simulink model "Part_3_Template"  (R2017a)
settings: Solver=ode3  StartTime=0.0  StopTime=30  FixedStep=.001  RelTol=1e-3  EnableMultiTasking=on
libraries: dspinverses x1
settings Model: Creator=Andrew Petruska  LastModifiedBy=siddh
settings OptimizationCC: LifeSpan=inf
settings DebuggingCC: SFUnexpectedBacktrackingDiag=warning  SFNoUnconditionalDefaultTransitionDiag=warning  SFExecutionAtInitializationDiag=none
settings GRTTargetCC: TargetLangStandard=C89/C90 (ANSI)  GeneratePreprocessorConditionals=Disable all
settings ConfigComp: CovMetricSettings=dw  CovHtmlReporting=on  CovSaveCumulativeToWorkspaceVar=on  CovSaveSingleToWorkspaceVar=on  CovExternalEMLEnable=off

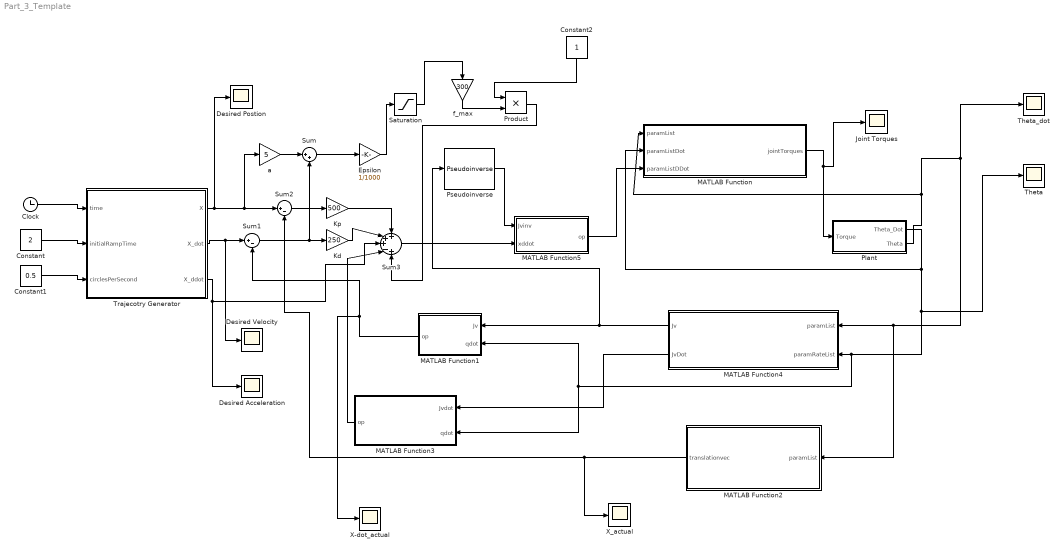
== system Part_3_Template ==
  Clock : Clock
  Constant : Constant  Value=2
  Constant1 : Constant  Value=0.5
  Constant2 : Constant
  Desired Acceleration : Scope
  Desired Postion : Scope
  Desired Velocity : Scope
  "Epsilon " : Gain  Gain=1/1000
  "Joint Torques " : Scope
  Kd : Gain  Gain=250
  Kp : Gain  Gain=500
  MATLAB Function : MATLAB Function  TreatAsAtomicUnit=on
  MATLAB Function1 : MATLAB Function  TreatAsAtomicUnit=on
  MATLAB Function2 : MATLAB Function  TreatAsAtomicUnit=on
  MATLAB Function3 : MATLAB Function  TreatAsAtomicUnit=on
  MATLAB Function4 : MATLAB Function  TreatAsAtomicUnit=on
  MATLAB Function5 : MATLAB Function  TreatAsAtomicUnit=on
  Plant : Subsystem
  Product : Product
  Pseudoinverse : dspinverses/Pseudoinverse  wanterr=off  SimulateUsing=Interpreted execution
      settings: SourceProductName=DSP System Toolbox  SourceProductBaseCode=DS
  Saturation : Saturate  UpperLimit=1  LowerLimit=-1
  Sum : Sum  Inputs=|++
  Sum1 : Sum  Inputs=|+-
  Sum2 : Sum  Inputs=|+-
  Sum3 : Sum  Inputs=+++-+
  "Theta " : Scope
  Theta_dot : Scope
  Trajecotry Generator : MATLAB Function  TreatAsAtomicUnit=on
  X-dot_actual : Scope
  X_actual : Scope
  "a " : Gain  Gain=5
  f_max : Gain  Gain=300
  wires:
  Plant/2(Theta) -> MATLAB Function2/1(paramList), MATLAB Function4/1(paramList), Theta_dot/1, MATLAB Function/1(paramList)
  Clock/1 -> Trajecotry Generator/1(time)
  Constant/1 -> Trajecotry Generator/2(initialRampTime)
  Constant1/1 -> Trajecotry Generator/3(circlesPerSecond)
  Trajecotry Generator/1(X) -> "a "/1, Sum2/1, Desired Postion/1
  Trajecotry Generator/2(X_dot) -> Sum1/1, Desired Velocity/1
  Trajecotry Generator/3(X_ddot) -> Sum3/3, Desired Acceleration/1
  Plant/1(Theta_Dot) -> MATLAB Function/2(paramListDot), MATLAB Function3/2(qdot), MATLAB Function1/2(qdot), MATLAB Function4/2(paramRateList), "Theta "/1
  MATLAB Function/1(jointTorques) -> "Joint Torques "/1, Plant/1(Torque)
  MATLAB Function4/2(JvDot) -> MATLAB Function3/1(Jvdot)
  MATLAB Function2/1(translationvec) -> X_actual/1, Sum2/2
  Sum2/1 -> Kp/1
  Kp/1 -> Sum3/1
  Sum1/1 -> Sum/2, Kd/1
  Kd/1 -> Sum3/2
  MATLAB Function3/1(op) -> Sum3/4
  MATLAB Function4/1(Jv) -> Pseudoinverse/1, MATLAB Function1/1(Jv)
  MATLAB Function1/1(op) -> X-dot_actual/1, Sum1/2
  Sum3/1 -> MATLAB Function5/2(xddot)
  Pseudoinverse/1 -> MATLAB Function5/1(Jvinv)
  MATLAB Function5/1(op) -> MATLAB Function/3(paramListDDot)
  "a "/1 -> Sum/1
  Sum/1 -> "Epsilon "/1
  "Epsilon "/1 -> Saturation/1
  Saturation/1 -> f_max/1
  f_max/1 -> Product/2
  Constant2/1 -> Product/1
  Product/1 -> Sum3/5

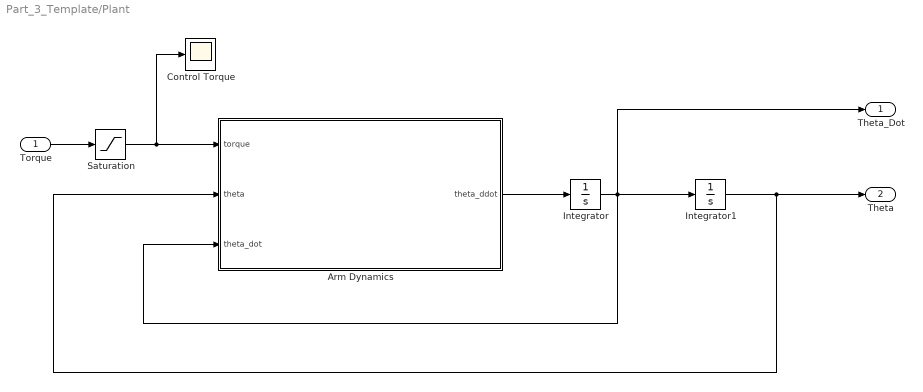
== system Part_3_Template/Plant ==
  Torque : Inport
  Arm Dynamics : MATLAB Function  TreatAsAtomicUnit=on
  Control Torque : Scope
  Integrator : Integrator  InitialCondition=[0;0;0]
  Integrator1 : Integrator  InitialCondition=[0;0;0]
  Saturation : Saturate  UpperLimit=300  LowerLimit=-300
  Theta_Dot : Outport
  Theta : Outport  Port=2
  wires:
  Torque/1 -> Saturation/1
  Arm Dynamics/1(theta_ddot) -> Integrator/1
  Integrator/1 -> Arm Dynamics/3(theta_dot), Integrator1/1, Theta_Dot/1
  Integrator1/1 -> Arm Dynamics/2(theta), Theta/1
  Saturation/1 -> Control Torque/1, Arm Dynamics/1(torque)

== matlab function Part_3_Template/Trajecotry Generator ==
  data: time input; X output; X_dot output; X_ddot output; initialRampTime input; circlesPerSecond input
function [X, X_dot, X_ddot] = fcn(time, initialRampTime, circlesPerSecond)
%#codegen

persistent a0 a1 a2 a3;

W = circlesPerSecond*2*pi;

if isempty(a0)
       
    t = initialRampTime;
    Ainv = [1,      0,     0,     0
        0,      0,     1,     0
        -3/t^2,  3/t^2,  -2/t,  -1/t
        2/t^3, -2/t^3, 1/t^2, 1/t^2];
    
    X0 = [1.5;0;0];
    Xf = X_t(0,W);
    V0 = [0;0;0];
    Vf = Xd_t(0,W);
    
    a0 = Ainv(1,1)*X0;
    a1 = Ainv(2,3)*V0;
    a2 = Ainv(3,1)*X0 + Ainv(3,2)*Xf + Ainv(3,3)*V0 +Ainv(3,4)*Vf;
    a3 = Ainv(4,1)*X0 + Ainv(4,2)*Xf + Ainv(4,3)*V0 +Ainv(4,4)*Vf;
    
end

if time <= initialRampTime
    X       = a0+a1*time+a2*time^2+a3*time^3;
    X_dot   = a1+2*a2*time+3*a3*time^2;
    X_ddot  = a2*2+6*a3*time;
else
    X = X_t(time-initialRampTime,W);
    X_dot = Xd_t(time-initialRampTime,W);
    X_ddot = Xdd_t(time-initialRampTime,W);
end

end

function xt = X_t(t,W)
%#codegen

xt = [.75+.5*sin(W*t);
      .5*cos(W*t);
      .5*sin(W*t)];
end

function xdt = Xd_t(t,W)
%#codegen

xdt = [.5*W*cos(W*t);
      -.5*W*sin(W*t);
       .5*W*cos(W*t)];
end

function xddt = Xdd_t(t,W)
%#codegen

xddt = [.5*W^2*sin(W*t);
    .5*W^2*cos(W*t);
    .5*W^2*sin(W*t)];
end

== matlab function Part_3_Template/Plant/Arm Dynamics ==
  data: torque input; theta_ddot output; theta input; theta_dot input
function theta_ddot = fcn(torque, theta, theta_dot)
%#codegen

% define physical parmaeters of the arm
density = 2.70e3;
 
r = 0.05;
L0 = 0.25;
L1 = 1;
L2 = .5;
 
m1 = density*(r^2*pi*L0);
m2 = density*(r^2*pi*L1);
m3 = density*(r^2*pi*L2);

cd = .5;
cs = 3;

g = 9.8;

% unpack theta and theta_dot
t1 = theta(1);
t2 = theta(2);
t3 = theta(3);

td1 = theta_dot(1);
td2 = theta_dot(2);
td3 = theta_dot(3);

% Define M(th)^-1, V(th,thdot), G(th) and F(th,th_dot)

theta_ddot = zeros(3,1);
theta_ddot = [ (24*torque(1) - 24*cd*td1 - 24*cs*sign(td1) - 6*m3*r^2*td1*td2*sin(2*t2 + 2*t3) - 6*m3*r^2*td1*td3*sin(2*t2 + 2*t3) + 8*L1^2*m2*td1*td2*sin(2*t2) + 24*L1^2*m3*td1*td2*sin(2*t2) - 6*m2*r^2*td1*td2*sin(2*t2) + 8*L2^2*m3*td1*td2*sin(2*t2 + 2*t3) + 8*L2^2*m3*td1*td3*sin(2*t2 + 2*t3) + 12*L1*L2*m3*td1*td3*sin(t3) + 24*L1*L2*m3*td1*td2*sin(2*t2 + t3) + 12*L1*L2*m3*td1*td3*sin(2*t2 + t3))/(4*L1^2*m2 + 12*L1^2*m3 + 4*L2^2*m3 + 12*m1*r^2 + 9*m2*r^2 + 9*m3*r^2 - 3*m3*r^2*cos(2*t2 + 2*t3) + 4*L1^2*m2*cos(2*t2) + 12*L1^2*m3*cos(2*t2) - 3*m2*r^2*cos(2*t2) + 4*L2^2*m3*cos(2*t2 + 2*t3) + 12*L1*L2*m3*cos(t3) + 12*L1*L2*m3*cos(2*t2 + t3));
 (cos(t3)*(72*L1*L2*cs*sign(td3) - 72*L1*L2*torque(3) + 72*L1*L2*cd*td3) + 48*L2^2*torque(2) - 48*L2^2*torque(3) + 36*r^2*torque(2) - 36*r^2*torque(3) - 36*cd*r^2*td2 - 48*L2^2*cs*sign(td2) - 36*cs*r^2*sign(td2) - 48*L2^2*cd*td2 + (9*m2*r^4*td1^2*sin(2*t2))/2 + 24*L1*L2^2*g*m2*cos(t2) + 30*L1*L2^2*g*m3*cos(t2) + 6*L1*L2^3*m3*td1^2*sin(2*t2 + 3*t3) + 18*L1*g*m2*r^2*cos(t2) + 36*L1*g*m3*r^2*cos(t2) - 18*L1*L2^2*g*m3*cos(t2 + 2*t3) - 8*L1^2*L2^2*m2*td1^2*sin(2*t2) - 15*L1^2*L2^2*m3*td1^2*sin(2*t2) + 9*L1^2*L2^2*m3*td1^2*sin(2*t3) + 18*L1^2*L2^2*m3*td2^2*sin(2*t3) - 6*L1^2*m2*r^2*td1^2*sin(2*t2) - 18*L1^2*m3*r^2*td1^2*sin(2*t2) + 6*L2^2*m2*r^2*td1^2*sin(2*t2) + 9*L1^2*L2^2*m3*td1^2*sin(2*t2 + 2*t3) + 12*L1*L2^3*m3*td1^2*sin(t3) + 24*L1*L2^3*m3*td2^2*sin(t3) + 24*L1*L2^3*m3*td3^2*sin(t3) - 6*L1*L2^3*m3*td1^2*sin(2*t2 + t3) - (27*L1*L2*m3*r^2*td1^2*sin(2*t2 + t3))/2 - (9*L1*L2*m3*r^2*td1^2*sin(2*t2 + 3*t3))/2 + 48*L1*L2^3*m3*td2*td3*sin(t3) + 9*L1*L2*m3*r^2*td1^2*sin(t3) + 18*L1*L2*m3*r^2*td2^2*sin(t3) + 18*L1*L2*m3*r^2*td3^2*sin(t3) + 36*L1*L2*m3*r^2*td2*td3*sin(t3))/(9*m2*r^4 + 16*L1^2*L2^2*m2 + 48*L1^2*L2^2*m3 + 12*L1^2*m2*r^2 + 36*L1^2*m3*r^2 + 12*L2^2*m2*r^2 - 36*L1^2*L2^2*m3*cos(t3)^2);
 - (12*(4*L2^2 + 6*L1*cos(t3)*L2 + 3*r^2)*(torque(2) - cd*td2 - cd*td3 - cs*sign(td2) - cs*sign(td3) + (L2*g*m3*cos(t2 + t3))/2 + (L1*g*m2*cos(t2))/2 + L1*g*m3*cos(t2) - (L1^2*m2*td1^2*sin(2*t2))/6 - (L1^2*m3*td1^2*sin(2*t2))/2 + (m2*r^2*td1^2*sin(2*t2))/8 - (L2^2*m3*td1^2*sin(2*t2 + 2*t3))/6 + (m3*r^2*td1^2*sin(2*t2 + 2*t3))/8 + (L1*L2*m3*td3^2*sin(t3))/2 - (L1*L2*m3*td1^2*sin(2*t2 + t3))/2 + L1*L2*m3*td2*td3*sin(t3)))/(9*m2*r^4 + 16*L1^2*L2^2*m2 + 48*L1^2*L2^2*m3 + 12*L1^2*m2*r^2 + 36*L1^2*m3*r^2 + 12*L2^2*m2*r^2 - 36*L1^2*L2^2*m3*cos(t3)^2) - ((48*L1^2*m2 + 144*L1^2*m3 + 48*L2^2*m3 + 36*m2*r^2 + 36*m3*r^2 + 144*L1*L2*m3*cos(t3))*(cd*td3 - torque(3) + cs*sign(td3) - (L2*g*m3*cos(t2 + t3))/2 + (L2^2*m3*td1^2*sin(2*t2 + 2*t3))/6 - (m3*r^2*td1^2*sin(2*t2 + 2*t3))/8 + (L1*L2*m3*td1^2*sin(t3))/4 + (L1*L2*m3*td2^2*sin(t3))/2 + (L1*L2*m3*td1^2*sin(2*t2 + t3))/4))/(m3*(9*m2*r^4 + 16*L1^2*L2^2*m2 + 48*L1^2*L2^2*m3 + 12*L1^2*m2*r^2 + 36*L1^2*m3*r^2 + 12*L2^2*m2*r^2 - 36*L1^2*L2^2*m3*cos(t3)^2))];
 
end

== matlab function Part_3_Template/MATLAB Function ==
  data: jointTorques output; paramList input; paramListDot input; paramListDDot input
% FUNCTION NAME : newtonEuler
% DESCRIPTION   : This function computes the inverse dynamics of a serial link manipulator
%                 and provides the velocity jacobian and its rate of change.
%
% OUTPUT        : The output gives the the joint torques at each joint,
%                 velocity Jacobian and time derivative of velocity
%                 Jacobian.
%
% INPUT         : The inputs are a list of joint parameters created
%                 with createLink,the the current joint angles/distances,
%                 the current joint angle/distance speeds,
%                 the current joint angle/distance accelerations and
%                 the boundary conditions corresponding to angular
%                 velocity, angular acceleration, linear acceleration,
%                 force and torque.
%
% NAME          : SIDDHARTH VISWANATHAN
% CWID          : 10831326
% COURSE NO.    : MEGN 544
% DATE          : 11/19/2017
%%
function jointTorques  = newtonEuler( paramList, paramListDot, paramListDDot )
% Intializing the values
N=3; 
a = zeros(N,1);
d = zeros(N,1);
alpha = zeros(N,1);
theta = zeros(N,1);
J_Inertia = zeros(3,3,N);
theta_dot = zeros(N,1);
theta_ddot = zeros(N,1);
d_dot = zeros(N,1);
d_ddot = zeros(N,1); 
J = zeros(3,3,N); 
rcom = zeros(3,N);
rcom_base = zeros(3,N);
m = zeros(N,1);
jointTorques = zeros(N,1);
li1=[0.03091,6.625e-3,0.03091];
li2=[0.0265,1.7799,1.7799];
li3=[0.01325,0.2275,0.2275];
linkList=repmat(createLink(0,0.25,pi/2,[],[0;-0.125;0],5.30,diag(li1)),[N,1]);
linkList(1)=createLink(0,0.25,pi/2,[],[0;-0.125;0],5.30,diag(li1));
linkList(2)=createLink(1,0,0,[],[-0.5;0;0],21.20,diag(li2));
linkList(3)=createLink(0.5,0,0,[],[-0.25;0;0],10.60,diag(li3));
boundary_conditions = struct('angV',zeros(3,1),'linA',zeros(3,1),'angA',zeros(3,1));
boundary_conditions.base_angular_velocity = [0;0;0];
boundary_conditions.base_linear_acceleration = [0;0;-9.8];
boundary_conditions.base_angular_acceleration= [0;0;0];
boundary_conditions.distal_force = [0;0;0];
boundary_conditions.distal_torque = [0;0;0];
T = zeros(4,4,N); 
dd = zeros(3,N+1);
Z = zeros(3,N+1); 
w = zeros(3,N+1); 
dd_dot = zeros(3,N+1);
H = eye(4);
w_dot = zeros(3,N+1);
dd_ddot = zeros(3,N+1);
rcom_base_dot = zeros(3,N);
rcom_base_ddot = zeros(3,N);
f = zeros(3,N+1);
n = zeros(3,N+1);
R=zeros(3,3,3);
%%
for i = 1:N
    a(i) = linkList(i).a;
    alpha(i) = linkList(i).alpha;
    d(i) = linkList(i).d;
    theta(i) = paramList(i);
    theta_dot(i) = paramListDot(i);
    theta_ddot(i) = paramListDDot(i);
    J_Inertia(:,:,i) = linkList(i).inertia;
    rcom(:,i) = linkList(i).com;
    m(i) = linkList(i).mass;
end
%%
for i = 1:N
    T(:,:,i) = zeros(4,4);
end
%%
dd(:,1) = [0; 0; 0];
Z(:,1) = [0; 0; 1];

for i = 1:N
    T(:,:,i)=H*dhTransform(a(i),d(i),alpha(i),theta(i));
    H = T(:,:,i);
end
%%
for i = 2:N+1
    dd(:,i) = T(1:3,4,i-1);
    Z(:,i) = T(1:3,3,i-1);
    R(:,:,i-1) = T(1:3,1:3,i-1);
end
%%
for i = 1:N
    J(:,:,i) = R(:,:,i)*J_Inertia(:,:,i)*R(:,:,i)';
end
%%
w(:,1) = boundary_conditions(1).base_angular_velocity;

for i = 2:N+1
        w(:,i) = w(:,i-1) + theta_dot(i-1)*Z(:,i-1);
end
%%
w_dot(:,1) = boundary_conditions(1).base_angular_acceleration;
w_dot(:,2) = w_dot(:,1) + theta_ddot(1)*Z(:,1) + cross(w(:,1),Z(:,1));

for i = 3:N+1
        w_dot(:,i) = w_dot(:,i-1) + theta_ddot(i-1)*Z(:,i-1) + cross(w(:,i-1),w(:,i));
end
%%
dd_dot(:,1) = [0; 0; 0];

for i = 2:N+1
        dd_dot(:,i) = dd_dot(:,i-1) + cross(w(:,i),(dd(:,i)-dd(:,i-1)));
end
%%
dd_ddot(:,1) = boundary_conditions(1).base_linear_acceleration;

for i = 2:N+1
        dd_ddot(:,i:i) = dd_ddot(:,i-1) + cross(w_dot(:,i),(dd(:,i)-dd(:,i-1))) + cross(w(:,i),cross(w(:,i),(dd(:,i)-dd(:,i-1))));
end
%%
for i = 1:N
    rcom_base(:,i) = R(:,:,i)*rcom(:,i);
end
%%
for i = 1:N
        rcom_base_dot(:,i) = dd_dot(:,i) + cross(w(:,i+1),rcom(:,i));
end
%%
for i = 1:N
        rcom_base_ddot(:,i) = dd_ddot(:,i) + cross(w_dot(:,i+1),(dd(:,i+1)-dd(:,i)+rcom_base(:,i))) + cross(w(:,i+1),cross(w(:,i+1),(dd(:,i+1)-dd(:,i)+rcom_base(:,i))));
end
%%
f(:,N+1) = boundary_conditions(1).distal_force;
n(:,N+1) = boundary_conditions(1).distal_torque;
%%
for i = N:-1:1
    
    f(:,i) = f(:,i+1) + m(i)*rcom_base_ddot(:,i);
    n(:,i) = n(:,i+1) + cross(dd(:,i+1)-dd(:,i)+rcom_base(:,i),f(:,i)) + J(:,:,i)*w_dot(:,i+1) + cross(w(:,i+1),J(:,:,i)*w(:,i+1)) - cross(rcom_base(:,i),f(:,i+1));
    jointTorques(i,1) = Z(:,i).'*n(:,i);
end
end

== matlab function Part_3_Template/MATLAB Function1 ==
  data: Jv input; op output; qdot input
function op = jvmultiply(Jv, qdot)
mult=Jv*qdot;
op=mult(1:3,1);
end

== matlab function Part_3_Template/MATLAB Function2 ==
  data: paramList input; translationvec output
% FUNCTION NAME : dhFwdKine 
% DESCRIPTION   : This function returns forward kinematics of a manipulator 
%                 with the provided DH parameter set. 
%
% OUTPUT        : The output gives a homogenous transform for the manipulator.
%
% INPUT         : The inputs are an array of links, each created by createLink
%                 and an array containing the current state of their joint variables.
%
% NAME          : SIDDHARTH VISWANATHAN
% CWID          : 10831326
% COURSE NO.    : MEGN 544
% DATE          : 11/19/2017
%%
function translationvec =dhFwdKine(paramList)
% Intializing values
translationvec=zeros(3,1);
noflinks= 3;
ht=zeros(4,4,3);
ab=zeros(4,4,3);
H=zeros(4,4,3);
li1=[0.03091,0.03091,6.625e-3];
li2=[0.0265,1.7799,1.7799];
li3=[0.01325,0.2275,0.2275];
linkList=repmat(createLink(0,0.25,pi/2,[],[0;0.125;0],5.30,diag(li1)),[noflinks,1]);
linkList(1)=createLink(0,0.25,pi/2,[],[0;0.125;0],5.30,diag(li1));
linkList(2)=createLink(1,0,0,[],[-0.5;0;0],21.20,diag(li2));
linkList(3)=createLink(0.5,0,0,[],[-0.5;0;0],10.60,diag(li3));
temp= linkList;
%%
% dH transform calculation for the links
for i= 1: noflinks             
          ht(:,:,i) = dhTransform(temp(i).a,temp(i).d,temp(i).alpha,paramList(i));
end
%%
% FIunding the final state of all links
for i = 1:noflinks-1           
   
    if i == 1
        ab = ht(:,:,1);
        H = ab*ht(:,:,2);
    else
        ab = H*ht(:,:,i+1);
        H = ab;
    end
    
end

translationvec=H(1:3,4);

end

== matlab function Part_3_Template/MATLAB Function3 ==
  data: Jvdot input; qdot input; op output
function op = jvdotmultiply(Jvdot, qdot)
mult=Jvdot*qdot;
op=mult(1:3,1);
end

== matlab function Part_3_Template/MATLAB Function4 ==
  data: Jv output; paramList input; paramRateList input; JvDot output
% FUNCTION NAME : velocityJacobian 
% DESCRIPTION   : This function returns the velocity jacobian of the manipulator 
%                 given an array of links created by the createLink function 
%                 and the current joint variables.
%
% OUTPUT        : The output gives velocity Jacobian and the time derivative of 
%                 velocity Jacobian.
%
% INPUT         : The inputs are a list of joint parameters created
%                 with createLink,the current theta or d values for the joints
%                 and  the current theta_dot and d_dot values for the joints.
%
% NAME          : SIDDHARTH VISWANATHAN
% CWID          : 10831326
% COURSE NO.    : MEGN 544
% DATE          : 11/19/2017
%%
function [Jv, JvDot] = velocityJacobian(paramList, paramRateList)
% Intializing the values
N=3;
a = zeros(N,1);
d = zeros(N,1);
alpha = zeros(N,1);
theta = zeros(N,1);
isRotary = zeros(N,1);
d_dot = zeros(N,1);
theta_dot = zeros(N,1);
T=zeros(4,4,N);
JvDot = zeros(6,3);
Jv=zeros(6,3);
li1=[0.03091,6.625e-3,0.03091];
li2=[0.0265,1.7799,1.7799];
li3=[0.01325,0.2275,0.2275];
linkList=repmat(createLink(0,0.25,pi/2,[],[0;-0.125;0],5.30,diag(li1)),[N,1]);
linkList(1)=createLink(0,0.25,pi/2,[],[0;-0.125;0],5.30,diag(li1));
linkList(2)=createLink(1,0,0,[],[-0.5;0;0],21.20,diag(li2));
linkList(3)=createLink(0.5,0,0,[],[-0.25;0;0],10.60,diag(li3));
dd = zeros(3,N+1);
Z = zeros(3,N+1);
w = zeros(3,N+1);
dd_dot = zeros(3,4);
H = eye(4);
%%
for i = 1:N
    a(i) = linkList(i).a;
    alpha(i) = linkList(i).alpha;
    d(i) = linkList(i).d;
    theta(i) = paramList(i);
    theta_dot(i) = paramRateList(i);
end
%%
for i = 1:N
    T(:,:,i) = zeros(4,4);
end
%%
for i = 1:N
    T(:,:,i)=H*dhTransform(a(i),d(i),alpha(i),theta(i));
    H = T(:,:,i);
end
%%
dd(:,1:1) = [0; 0; 0];
Z(:,1) = [0 0 1];
w(:,1:1) = [0; 0; 0];
dd_dot(:,1:1) = [0; 0; 0];
for i = 2:N+1
    dd(:,i:i) =  T(1:3,4:4,i-1);
    Z(:,i) = T(1:3,3:3,i-1);
    if isRotary(i-1) == 1
        w(:,i) = theta_dot(i-1)*Z(:,i-1)+w(:,i-1);
    else
        w(:,i) = w(:,i-1);
    end
    if isRotary(i-1) == 1
        dd_dot(:,i) = dd_dot(:,i-1) + cross(w(:,i),(dd(:,i)-dd(:,i-1)));
    else
        dd_dot(:,i) = dd_dot(:,i-1) + cross(w(:,i),(dd(:,i)-dd(:,i-1))) + d_dot(i-1)*Z(:,i-1);
    end
end
%% Velocity Jacobain
for i = 1:N
        Jv(1:3,i) = cpMap(Z(:,i))*(T(1:3,4,N)-dd(:,i));
        Jv(4:6,i) = Z(:,i);
end
%% Velcoity hessian (Jv_dot)
for i = 1:N
        JvDot(:,i) = [cross(cross(w(:,i),Z(:,i)),(dd(:,N+1)-dd(:,i)))+cross(Z(:,i),dd_dot(:,4)-dd_dot(:,i)); cross(w(:,i),Z(:,i))];
end​
end

== matlab function Part_3_Template/MATLAB Function5 ==
  data: Jvinv input; op output; xddot input
function op =jvinverse(Jvinv,xddot)
Jvinv1=Jvinv(1:3,1:3);
op=Jvinv1*xddot;
end
